simulink model "cubli_XYZ_extensive_simulations"  (R2016a)
settings: Solver=VariableStepAuto  StartTime=0.0  StopTime=10  FixedStep=0.001  RelTol=1e-3
values from neighbouring files (symbols this model uses):
  a = 0.15    [init.m]
  M = 2.5    [init.m]    (also in skew.m = [0 -z y)
  m = 0.204    [init.m]
  s = size(delta_i)    [accessibility_test.m]    (also in observability_test.m = size(delta_i,1))
  state0 = get_equilibrium(0, -pi/4, pi/2, f, state)    [init.m]
undefined symbols (not defined in the file or in its folder): X, Y, Z
libraries: sm_lib x15, nesl_utility x13
(part 2 of 9)

== matlab function cubli_XYZ_extensive_simulations/Cubli/Controller/noninteractive feedback control ==
  data: v input; state input; u output
 function u = nic_fnc(v, state)

th1 = state(1);
th2 = state(2);
th3 = state(3);

th1dot = state(4);
th2dot = state(5);
th3dot = state(6);
qxdot = state(7);
qydot = state(8);
qzdot = state(9);

A = [                                                                                                                  -(11529215046068469760000*(173808361171031714041*cos(th3) - 97421867139278569472*sin(th3)))/(50688073959935957106266099682798465939237*cos(th2)*(cos(th3)^2 + sin(th3)^2)),                                                                                                                  -(11529215046068469760000*(97421867139278569472*cos(th3) - 173808361171031714041*sin(th3)))/(50688073959935957106266099682798465939237*cos(th2)*(cos(th3)^2 + sin(th3)^2)),                                                                                                                                          -(1123197656438253912603716965936891166720000*(cos(th3) - sin(th3)))/(50688073959935957106266099682798465939237*cos(th2)*(cos(th3)^2 + sin(th3)^2))
                                                                                                                           -(11529215046068469760000*(97421867139278569472*cos(th3) + 173808361171031714041*sin(th3)))/(50688073959935957106266099682798465939237*(cos(th3)^2 + sin(th3)^2)),                                                                                                                           -(11529215046068469760000*(173808361171031714041*cos(th3) + 97421867139278569472*sin(th3)))/(50688073959935957106266099682798465939237*(cos(th3)^2 + sin(th3)^2)),                                                                                                                                                   -(1123197656438253912603716965936891166720000*(cos(th3) + sin(th3)))/(50688073959935957106266099682798465939237*(cos(th3)^2 + sin(th3)^2))
 -(11529215046068469760000*(97421867139278569472*sin(th2)*sin(th3) - 173808361171031714041*cos(th3)*sin(th2) + 97421867139278569472*cos(th2)*cos(th3)^2 + 97421867139278569472*cos(th2)*sin(th3)^2))/(50688073959935957106266099682798465939237*(cos(th2)*cos(th3)^2 + cos(th2)*sin(th3)^2)), -(11529215046068469760000*(173808361171031714041*sin(th2)*sin(th3) - 97421867139278569472*cos(th3)*sin(th2) + 97421867139278569472*cos(th2)*cos(th3)^2 + 97421867139278569472*cos(th2)*sin(th3)^2))/(50688073959935957106266099682798465939237*(cos(th2)*cos(th3)^2 + cos(th2)*sin(th3)^2)), -(11529215046068469760000*(97421867139278569472*sin(th2)*sin(th3) - 97421867139278569472*cos(th3)*sin(th2) + 173808361171031714041*cos(th2)*cos(th3)^2 + 173808361171031714041*cos(th2)*sin(th3)^2))/(50688073959935957106266099682798465939237*(cos(th2)*cos(th3)^2 + cos(th2)*sin(th3)^2))];
 
b = [                                                                                                                                                                                                                                                                                                                                                                                                                                                                                                                                                                                                                                                                                                                                                                                                                                                                                                                                                                                                                                                                                                                                                                                                                                                                                                                                                                                                                                                                                                                                                                                                                                                                                                                                                                                                                                                                                                                                                                                                                                                                                                                                                                                                                                                                                                                                                                                                                                                                                                                                                                                                                                                                                                                                                                                                                                                                                                                                                                                                                                                                                                                                                                                                                                                                                                                                                                                                                                                                                                                                                                                                                                                                                                                                                                                                                                                                                                                                                                                                                                                                                                                                                                                                                                                                                                                                                                                                                                                                                                                                                                                                                                                                                                                                                                                                                                                                                                                                                                                                                                                                                                                                                                                                                                                                                                                                                                                                                                                                                                                                                                                                                                                                                                                                                                                                                                                                                                                                                                                                                                                                                                                                                                                                                                                                                                                                                                                                                                                                                                                                                                                                                                                                                                                                                                                                                                                                                                                                                                                                                                                                                                                                                                                                                                                                                                                                                                                                                                                                                                                                                                                                                                                                                                                                                                                                                                                                                                                                                                                                                                                                                                                                                                                                                                                                                                                                                                                                                                                                                                                                                                                                                                                                                                                                                                                           -(11909473891670740540090329827195917399228416*cos(th1)*cos(th3)^3 + 11909473891670740540090329827195917399228416*cos(th1)*sin(th3)^3 - 84663675348499979021291712024873281781760*th2dot^2*cos(th2)*cos(th3)^3 + 37208574363983751213784670214039629987840*th3dot^2*cos(th2)*cos(th3)^3 + 47455100984516227807507041810833651793920*th2dot^2*cos(th2)*cos(th3)^5 - 84663675348499979021291712024873281781760*th2dot^2*cos(th2)*sin(th3)^3 + 37208574363983751213784670214039629987840*th3dot^2*cos(th2)*sin(th3)^3 + 47455100984516227807507041810833651793920*th2dot^2*cos(th2)*sin(th3)^5 - 11909473891670740540090329827195917399228416*cos(th2)*cos(th3)^2*sin(th1) - 1441358891699742679378121702564642609430528*cos(th1)*cos(th3)*sin(th3)^2 - 1441358891699742679378121702564642609430528*cos(th1)*cos(th3)^2*sin(th3) + 6675416391685241609734225764880280004329472*cos(th2)*cos(th3)^4*sin(th1) - 11909473891670740540090329827195917399228416*cos(th2)*sin(th1)*sin(th3)^2 + 6675416391685241609734225764880280004329472*cos(th2)*sin(th1)*sin(th3)^4 + 47455100984516227807507041810833651793920*th1dot^2*cos(th2)^3*cos(th3)^3 - 47455100984516227807507041810833651793920*th1dot^2*cos(th2)^3*cos(th3)^5 - 6675416391685241609734225764880280004329472*cos(th1)*cos(th2)^2*cos(th3)^3 + 47455100984516227807507041810833651793920*th1dot^2*cos(th2)^3*sin(th3)^3 - 47455100984516227807507041810833651793920*th1dot^2*cos(th2)^3*sin(th3)^5 - 6675416391685241609734225764880280004329472*cos(th1)*cos(th2)^2*sin(th3)^3 - 11909473891670740540090329827195917399228416*cos(th1)*cos(th3)^3*sin(th2)^2 - 11909473891670740540090329827195917399228416*cos(th1)*sin(th2)^2*sin(th3)^3 + 10246526620532476593722371596794021806080*th2dot^2*cos(th2)*cos(th3)*sin(th3)^2 + 10246526620532476593722371596794021806080*th2dot^2*cos(th2)*cos(th3)^2*sin(th3) + 37208574363983751213784670214039629987840*th3dot^2*cos(th2)*cos(th3)*sin(th3)^2 + 37208574363983751213784670214039629987840*th3dot^2*cos(th2)*cos(th3)^2*sin(th3) - 47455100984516227807507041810833651793920*th2dot^2*cos(th2)*cos(th3)*sin(th3)^4 - 47455100984516227807507041810833651793920*th2dot^2*cos(th2)*cos(th3)^4*sin(th3) - 6675416391685241609734225764880280004329472*cos(th1)*cos(th2)*cos(th3)^2*sin(th2) + 6675416391685241609734225764880280004329472*cos(th1)*cos(th2)*cos(th3)^4*sin(th2) + 6675416391685241609734225764880280004329472*cos(th1)*cos(th2)*sin(th2)*sin(th3)^2 - 6675416391685241609734225764880280004329472*cos(th1)*cos(th2)*sin(th2)*sin(th3)^4 - 13350832783370483219468451529760560008658944*cos(th2)*cos(th3)*sin(th1)*sin(th3)^3 - 13350832783370483219468451529760560008658944*cos(th2)*cos(th3)^3*sin(th1)*sin(th3) - 795598339977096578581794905915392000000*qxdot*th2dot*cos(th2)*cos(th3)^4 + 795598339977096578581794905915392000000*qxdot*th3dot*cos(th2)*cos(th3)^3 - 1419410730694772925795933922925238500000*qydot*th3dot*cos(th2)*cos(th3)^3 + 1419410730694772925795933922925238500000*qzdot*th2dot*cos(th2)*cos(th3)^2 + 237129818143993776058215849996810503030165*th2dot*th3dot*cos(th2)*cos(th3)^2 - 96329612699727228540810017544592542087840*th2dot*th3dot*cos(th2)*cos(th3)^4 - 1419410730694772925795933922925238500000*qxdot*th3dot*cos(th2)*sin(th3)^3 - 795598339977096578581794905915392000000*qydot*th2dot*cos(th2)*sin(th3)^4 + 795598339977096578581794905915392000000*qydot*th3dot*cos(th2)*sin(th3)^3 + 1419410730694772925795933922925238500000*qzdot*th2dot*cos(th2)*sin(th3)^2 + 237129818143993776058215849996810503030165*th2dot*th3dot*cos(th2)*sin(th3)^2 - 96329612699727228540810017544592542087840*th2dot*th3dot*cos(th2)*sin(th3)^4 - 132914374672993303407380548741622325575680*th1dot^2*cos(th2)^2*cos(th3)^2*sin(th2) + 37208574363983751213784670214039629987840*th1dot^2*cos(th2)*cos(th3)^3*sin(th2)^2 + 170122949036977054621165218955661955563520*th1dot^2*cos(th2)^2*cos(th3)^4*sin(th2) - 47455100984516227807507041810833651793920*th1dot^2*cos(th2)^3*cos(th3)*sin(th3)^2 - 47455100984516227807507041810833651793920*th1dot^2*cos(th2)^3*cos(th3)^2*sin(th3) + 47455100984516227807507041810833651793920*th1dot^2*cos(th2)^3*cos(th3)*sin(th3)^4 + 47455100984516227807507041810833651793920*th1dot^2*cos(th2)^3*cos(th3)^4*sin(th3) + 6675416391685241609734225764880280004329472*cos(th1)*cos(th2)^2*cos(th3)*sin(th3)^2 + 6675416391685241609734225764880280004329472*cos(th1)*cos(th2)^2*cos(th3)^2*sin(th3) + 132914374672993303407380548741622325575680*th1dot^2*cos(th2)^2*sin(th2)*sin(th3)^2 + 37208574363983751213784670214039629987840*th1dot^2*cos(th2)*sin(th2)^2*sin(th3)^3 - 170122949036977054621165218955661955563520*th1dot^2*cos(th2)^2*sin(th2)*sin(th3)^4 + 1441358891699742679378121702564642609430528*cos(th1)*cos(th3)*sin(th2)^2*sin(th3)^2 + 1441358891699742679378121702564642609430528*cos(th1)*cos(th3)^2*sin(th2)^2*sin(th3) + 13350832783370483219468451529760560008658944*cos(th2)*cos(th3)^2*sin(th1)*sin(th3)^2 + 795598339977096578581794905915392000000*qydot*th1dot*cos(th2)^2*cos(th3)^4 - 795598339977096578581794905915392000000*qzdot*th1dot*cos(th2)^2*cos(th3)^2 - 37208574363983751213784670214039629987840*th1dot*th2dot*cos(th2)^2*cos(th3)^3 - 132914374672993303407380548741622325575680*th1dot*th3dot*cos(th2)^2*cos(th3)^2 + 170122949036977054621165218955661955563520*th1dot*th3dot*cos(th2)^2*cos(th3)^4 - 795598339977096578581794905915392000000*qxdot*th1dot*cos(th2)^2*sin(th3)^4 + 795598339977096578581794905915392000000*qzdot*th1dot*cos(th2)^2*sin(th3)^2 + 37208574363983751213784670214039629987840*th1dot*th2dot*cos(th2)^2*sin(th3)^3 + 132914374672993303407380548741622325575680*th1dot*th3dot*cos(th2)^2*sin(th3)^2 - 170122949036977054621165218955661955563520*th1dot*th3dot*cos(th2)^2*sin(th3)^4 + 13350832783370483219468451529760560008658944*cos(th2)*cos(th3)*sin(th1)*sin(th3) + 795598339977096578581794905915392000000*qxdot*th1dot*cos(th2)*cos(th3)^3*sin(th2) + 795598339977096578581794905915392000000*qxdot*th2dot*cos(th2)*cos(th3)*sin(th3)^3 + 795598339977096578581794905915392000000*qxdot*th2dot*cos(th2)*cos(th3)^3*sin(th3) + 795598339977096578581794905915392000000*qxdot*th3dot*cos(th2)*cos(th3)*sin(th3)^2 - 1419410730694772925795933922925238500000*qxdot*th3dot*cos(th2)*cos(th3)^2*sin(th3) - 1419410730694772925795933922925238500000*qydot*th1dot*cos(th2)*cos(th3)^3*sin(th2) + 795598339977096578581794905915392000000*qydot*th2dot*cos(th2)*cos(th3)*sin(th3)^3 + 795598339977096578581794905915392000000*qydot*th2dot*cos(th2)*cos(th3)^3*sin(th3) - 1419410730694772925795933922925238500000*qydot*th3dot*cos(th2)*cos(th3)*sin(th3)^2 + 795598339977096578581794905915392000000*qydot*th3dot*cos(th2)*cos(th3)^2*sin(th3) + 237129818143993776058215849996810503030165*th1dot*th2dot*cos(th2)*cos(th3)^2*sin(th2) - 377930023588260323575621682449028463972490*th1dot*th2dot*cos(th2)*cos(th3)^4*sin(th2) + 74417148727967502427569340428079259975680*th1dot*th3dot*cos(th2)*cos(th3)^3*sin(th2) + 340245898073954109242330437911323911127040*th2dot*th3dot*cos(th2)*cos(th3)*sin(th3)^3 + 340245898073954109242330437911323911127040*th2dot*th3dot*cos(th2)*cos(th3)^3*sin(th3) - 1419410730694772925795933922925238500000*qxdot*th1dot*cos(th2)*sin(th2)*sin(th3)^3 + 795598339977096578581794905915392000000*qydot*th1dot*cos(th2)*sin(th2)*sin(th3)^3 + 237129818143993776058215849996810503030165*th1dot*th2dot*cos(th2)*sin(th2)*sin(th3)^2 - 377930023588260323575621682449028463972490*th1dot*th2dot*cos(th2)*sin(th2)*sin(th3)^4 + 74417148727967502427569340428079259975680*th1dot*th3dot*cos(th2)*sin(th2)*sin(th3)^3 + 37208574363983751213784670214039629987840*th1dot^2*cos(th2)*cos(th3)*sin(th2)^2*sin(th3)^2 + 37208574363983751213784670214039629987840*th1dot^2*cos(th2)*cos(th3)^2*sin(th2)^2*sin(th3) + 795598339977096578581794905915392000000*qxdot*th1dot*cos(th2)^2*cos(th3)*sin(th3)^3 + 795598339977096578581794905915392000000*qxdot*th1dot*cos(th2)^2*cos(th3)^3*sin(th3) - 795598339977096578581794905915392000000*qxdot*th2dot*cos(th2)*cos(th3)^2*sin(th3)^2 - 795598339977096578581794905915392000000*qydot*th1dot*cos(th2)^2*cos(th3)*sin(th3)^3 - 795598339977096578581794905915392000000*qydot*th1dot*cos(th2)^2*cos(th3)^3*sin(th3) - 795598339977096578581794905915392000000*qydot*th2dot*cos(th2)*cos(th3)^2*sin(th3)^2 - 227028978302048662443812837457374237163520*th1dot*th2dot*cos(th2)^2*cos(th3)*sin(th3)^2 + 227028978302048662443812837457374237163520*th1dot*th2dot*cos(th2)^2*cos(th3)^2*sin(th3) + 189820403938064911230028167243334607175680*th1dot*th2dot*cos(th2)^2*cos(th3)*sin(th3)^4 - 189820403938064911230028167243334607175680*th1dot*th2dot*cos(th2)^2*cos(th3)^4*sin(th3) - 192659225399454457081620035089185084175680*th2dot*th3dot*cos(th2)*cos(th3)^2*sin(th3)^2 - 1591196679954193157163589811830784000000*qzdot*th2dot*cos(th2)*cos(th3)*sin(th3) - 265828749345986606814761097483244651151360*th2dot*th3dot*cos(th2)*cos(th3)*sin(th3) - 795598339977096578581794905915392000000*qxdot*th1dot*cos(th2)^2*cos(th3)^2*sin(th3)^2 + 795598339977096578581794905915392000000*qydot*th1dot*cos(th2)^2*cos(th3)^2*sin(th3)^2 - 189820403938064911230028167243334607175680*th1dot*th2dot*cos(th2)^2*cos(th3)^2*sin(th3)^3 + 189820403938064911230028167243334607175680*th1dot*th2dot*cos(th2)^2*cos(th3)^3*sin(th3)^2 + 795598339977096578581794905915392000000*qxdot*th1dot*cos(th2)*cos(th3)*sin(th2)*sin(th3)^2 - 1419410730694772925795933922925238500000*qxdot*th1dot*cos(th2)*cos(th3)^2*sin(th2)*sin(th3) - 1419410730694772925795933922925238500000*qydot*th1dot*cos(th2)*cos(th3)*sin(th2)*sin(th3)^2 + 795598339977096578581794905915392000000*qydot*th1dot*cos(th2)*cos(th3)^2*sin(th2)*sin(th3) + 340245898073954109242330437911323911127040*th1dot*th2dot*cos(th2)*cos(th3)*sin(th2)*sin(th3)^3 + 340245898073954109242330437911323911127040*th1dot*th2dot*cos(th2)*cos(th3)^3*sin(th2)*sin(th3) + 74417148727967502427569340428079259975680*th1dot*th3dot*cos(th2)*cos(th3)*sin(th2)*sin(th3)^2 + 74417148727967502427569340428079259975680*th1dot*th3dot*cos(th2)*cos(th3)^2*sin(th2)*sin(th3) - 755860047176520647151243364898056927944980*th1dot*th2dot*cos(th2)*cos(th3)^2*sin(th2)*sin(th3)^2 - 265828749345986606814761097483244651151360*th1dot*th2dot*cos(th2)*cos(th3)*sin(th2)*sin(th3))/(140800205444266547517405832452217960942325*cos(th2)*(cos(th2)*cos(th3)^2 + cos(th2)*sin(th3)^2)*(cos(th3)^2 + sin(th3)^2))
                                                                                                                                                                                                                                                                                                                                                                                                                                                                                                                                                                                                                                                                                                                                                                                                                                                                                                                                                                                                                                                                                                                                                                                                                                                                                                                                                                                                                                                                                                                                                                                                                                                                                                                                                                                                                                                                                                                                                                                                                                                                                                                                                                                                                                                                                                                                                                                                                                                                                                                                                                                                                                                                                                                                                                                                                                                                                                                                                                                                                                                                                                                                                                                                                                                                                                                                                                                                                                                                                                                                                                                                                                                                                                                                                                                                                                                                                                                                                                                                                                                                                                                                                                                                                                                                                                                                                                                                                                                                                                                                                                                                                                                                                                                                                                                                                                                                                                                                                                                                                                                                                                                                                                                                                                                                                                                                                                                                                                                                                                                                                                                                                                                                                                                                                                                                                                                                                                                                                                                                                                                                                                                                                                                                                                                                                                                                                                                                                                                                                                                                                                                                                                                                                                                                                                                                                                                                                                                                                                                                                                                                                                                                                                                                                                                                                                                                                                                                                                                                                                                                                                                                                                                                                                                                                                                                                                                                                                                                                                                                                                                                                                                                                                                                                                                                                                                                                                                                                                                                                                                                                                                                                                                                                                                                                                    -(6675416391685241609734225764880280004329472*cos(th1)*cos(th3)^3 - 6675416391685241609734225764880280004329472*cos(th1)*sin(th3)^3 - 47455100984516227807507041810833651793920*th2dot^2*cos(th2)*cos(th3)^3 - 37208574363983751213784670214039629987840*th3dot^2*cos(th2)*cos(th3)^3 + 47455100984516227807507041810833651793920*th2dot^2*cos(th2)*cos(th3)^5 + 47455100984516227807507041810833651793920*th2dot^2*cos(th2)*sin(th3)^3 + 37208574363983751213784670214039629987840*th3dot^2*cos(th2)*sin(th3)^3 - 47455100984516227807507041810833651793920*th2dot^2*cos(th2)*sin(th3)^5 - 6675416391685241609734225764880280004329472*cos(th2)*cos(th3)^2*sin(th1) - 6675416391685241609734225764880280004329472*cos(th1)*cos(th3)*sin(th3)^2 + 6675416391685241609734225764880280004329472*cos(th1)*cos(th3)^2*sin(th3) + 6675416391685241609734225764880280004329472*cos(th2)*cos(th3)^4*sin(th1) + 6675416391685241609734225764880280004329472*cos(th2)*sin(th1)*sin(th3)^2 - 6675416391685241609734225764880280004329472*cos(th2)*sin(th1)*sin(th3)^4 + 84663675348499979021291712024873281781760*th1dot^2*cos(th2)^3*cos(th3)^3 - 47455100984516227807507041810833651793920*th1dot^2*cos(th2)^3*cos(th3)^5 - 11909473891670740540090329827195917399228416*cos(th1)*cos(th2)^2*cos(th3)^3 - 84663675348499979021291712024873281781760*th1dot^2*cos(th2)^3*sin(th3)^3 + 47455100984516227807507041810833651793920*th1dot^2*cos(th2)^3*sin(th3)^5 + 11909473891670740540090329827195917399228416*cos(th1)*cos(th2)^2*sin(th3)^3 - 6675416391685241609734225764880280004329472*cos(th1)*cos(th3)^3*sin(th2)^2 + 6675416391685241609734225764880280004329472*cos(th1)*sin(th2)^2*sin(th3)^3 + 47455100984516227807507041810833651793920*th2dot^2*cos(th2)*cos(th3)*sin(th3)^2 - 47455100984516227807507041810833651793920*th2dot^2*cos(th2)*cos(th3)^2*sin(th3) - 37208574363983751213784670214039629987840*th3dot^2*cos(th2)*cos(th3)*sin(th3)^2 + 37208574363983751213784670214039629987840*th3dot^2*cos(th2)*cos(th3)^2*sin(th3) - 47455100984516227807507041810833651793920*th2dot^2*cos(th2)*cos(th3)*sin(th3)^4 + 47455100984516227807507041810833651793920*th2dot^2*cos(th2)*cos(th3)^4*sin(th3) - 11909473891670740540090329827195917399228416*cos(th1)*cos(th2)*cos(th3)^2*sin(th2) + 6675416391685241609734225764880280004329472*cos(th1)*cos(th2)*cos(th3)^4*sin(th2) - 11909473891670740540090329827195917399228416*cos(th1)*cos(th2)*sin(th2)*sin(th3)^2 + 6675416391685241609734225764880280004329472*cos(th1)*cos(th2)*sin(th2)*sin(th3)^4 - 795598339977096578581794905915392000000*qxdot*th2dot*cos(th2)*cos(th3)^4 + 1419410730694772925795933922925238500000*qxdot*th3dot*cos(th2)*cos(th3)^3 - 795598339977096578581794905915392000000*qydot*th3dot*cos(th2)*cos(th3)^3 + 795598339977096578581794905915392000000*qzdot*th2dot*cos(th2)*cos(th3)^2 + 132914374672993303407380548741622325575680*th2dot*th3dot*cos(th2)*cos(th3)^2 - 170122949036977054621165218955661955563520*th2dot*th3dot*cos(th2)*cos(th3)^4 + 795598339977096578581794905915392000000*qxdot*th3dot*cos(th2)*sin(th3)^3 + 795598339977096578581794905915392000000*qydot*th2dot*cos(th2)*sin(th3)^4 - 1419410730694772925795933922925238500000*qydot*th3dot*cos(th2)*sin(th3)^3 - 795598339977096578581794905915392000000*qzdot*th2dot*cos(th2)*sin(th3)^2 - 132914374672993303407380548741622325575680*th2dot*th3dot*cos(th2)*sin(th3)^2 + 170122949036977054621165218955661955563520*th2dot*th3dot*cos(th2)*sin(th3)^4 - 237129818143993776058215849996810503030165*th1dot^2*cos(th2)^2*cos(th3)^2*sin(th2) - 37208574363983751213784670214039629987840*th1dot^2*cos(th2)*cos(th3)^3*sin(th2)^2 + 237129818143993776058215849996810503030165*th1dot^2*cos(th2)^2*cos(th3)^4*sin(th2) - 10246526620532476593722371596794021806080*th1dot^2*cos(th2)^3*cos(th3)*sin(th3)^2 + 10246526620532476593722371596794021806080*th1dot^2*cos(th2)^3*cos(th3)^2*sin(th3) + 47455100984516227807507041810833651793920*th1dot^2*cos(th2)^3*cos(th3)*sin(th3)^4 - 47455100984516227807507041810833651793920*th1dot^2*cos(th2)^3*cos(th3)^4*sin(th3) + 1441358891699742679378121702564642609430528*cos(th1)*cos(th2)^2*cos(th3)*sin(th3)^2 - 1441358891699742679378121702564642609430528*cos(th1)*cos(th2)^2*cos(th3)^2*sin(th3) - 237129818143993776058215849996810503030165*th1dot^2*cos(th2)^2*sin(th2)*sin(th3)^2 + 37208574363983751213784670214039629987840*th1dot^2*cos(th2)*sin(th2)^2*sin(th3)^3 + 237129818143993776058215849996810503030165*th1dot^2*cos(th2)^2*sin(th2)*sin(th3)^4 + 6675416391685241609734225764880280004329472*cos(th1)*cos(th3)*sin(th2)^2*sin(th3)^2 - 6675416391685241609734225764880280004329472*cos(th1)*cos(th3)^2*sin(th2)^2*sin(th3) + 795598339977096578581794905915392000000*qydot*th1dot*cos(th2)^2*cos(th3)^4 - 1419410730694772925795933922925238500000*qzdot*th1dot*cos(th2)^2*cos(th3)^2 + 37208574363983751213784670214039629987840*th1dot*th2dot*cos(th2)^2*cos(th3)^3 - 237129818143993776058215849996810503030165*th1dot*th3dot*cos(th2)^2*cos(th3)^2 + 96329612699727228540810017544592542087840*th1dot*th3dot*cos(th2)^2*cos(th3)^4 + 795598339977096578581794905915392000000*qxdot*th1dot*cos(th2)^2*sin(th3)^4 - 1419410730694772925795933922925238500000*qzdot*th1dot*cos(th2)^2*sin(th3)^2 + 37208574363983751213784670214039629987840*th1dot*th2dot*cos(th2)^2*sin(th3)^3 - 237129818143993776058215849996810503030165*th1dot*th3dot*cos(th2)^2*sin(th3)^2 + 96329612699727228540810017544592542087840*th1dot*th3dot*cos(th2)^2*sin(th3)^4 - 265828749345986606814761097483244651151360*th1dot^2*cos(th2)^2*cos(th3)*sin(th2)*sin(th3) + 13350832783370483219468451529760560008658944*cos(th1)*cos(th2)*cos(th3)*sin(th2)*sin(th3)^3 + 13350832783370483219468451529760560008658944*cos(th1)*cos(th2)*cos(th3)^3*sin(th2)*sin(th3) + 1419410730694772925795933922925238500000*qxdot*th1dot*cos(th2)*cos(th3)^3*sin(th2) - 795598339977096578581794905915392000000*qxdot*th2dot*cos(th2)*cos(th3)*sin(th3)^3 - 795598339977096578581794905915392000000*qxdot*th2dot*cos(th2)*cos(th3)^3*sin(th3) + 1419410730694772925795933922925238500000*qxdot*th3dot*cos(th2)*cos(th3)*sin(th3)^2 + 795598339977096578581794905915392000000*qxdot*th3dot*cos(th2)*cos(th3)^2*sin(th3) - 795598339977096578581794905915392000000*qydot*th1dot*cos(th2)*cos(th3)^3*sin(th2) + 795598339977096578581794905915392000000*qydot*th2dot*cos(th2)*cos(th3)*sin(th3)^3 + 795598339977096578581794905915392000000*qydot*th2dot*cos(th2)*cos(th3)^3*sin(th3) - 795598339977096578581794905915392000000*qydot*th3dot*cos(th2)*cos(th3)*sin(th3)^2 - 1419410730694772925795933922925238500000*qydot*th3dot*cos(th2)*cos(th3)^2*sin(th3) - 1591196679954193157163589811830784000000*qzdot*th1dot*cos(th2)^2*cos(th3)*sin(th3) + 132914374672993303407380548741622325575680*th1dot*th2dot*cos(th2)*cos(th3)^2*sin(th2) - 170122949036977054621165218955661955563520*th1dot*th2dot*cos(th2)*cos(th3)^4*sin(th2) - 74417148727967502427569340428079259975680*th1dot*th3dot*cos(th2)*cos(th3)^3*sin(th2) - 265828749345986606814761097483244651151360*th1dot*th3dot*cos(th2)^2*cos(th3)*sin(th3) + 795598339977096578581794905915392000000*qxdot*th1dot*cos(th2)*sin(th2)*sin(th3)^3 - 1419410730694772925795933922925238500000*qydot*th1dot*cos(th2)*sin(th2)*sin(th3)^3 - 132914374672993303407380548741622325575680*th1dot*th2dot*cos(th2)*sin(th2)*sin(th3)^2 + 170122949036977054621165218955661955563520*th1dot*th2dot*cos(th2)*sin(th2)*sin(th3)^4 + 74417148727967502427569340428079259975680*th1dot*th3dot*cos(th2)*sin(th2)*sin(th3)^3 - 37208574363983751213784670214039629987840*th1dot^2*cos(th2)*cos(th3)*sin(th2)^2*sin(th3)^2 + 37208574363983751213784670214039629987840*th1dot^2*cos(th2)*cos(th3)^2*sin(th2)^2*sin(th3) + 340245898073954109242330437911323911127040*th1dot^2*cos(th2)^2*cos(th3)*sin(th2)*sin(th3)^3 + 340245898073954109242330437911323911127040*th1dot^2*cos(th2)^2*cos(th3)^3*sin(th2)*sin(th3) + 13350832783370483219468451529760560008658944*cos(th1)*cos(th2)*cos(th3)^2*sin(th2)*sin(th3)^2 + 795598339977096578581794905915392000000*qxdot*th1dot*cos(th2)^2*cos(th3)*sin(th3)^3 + 795598339977096578581794905915392000000*qxdot*th1dot*cos(th2)^2*cos(th3)^3*sin(th3) - 795598339977096578581794905915392000000*qxdot*th2dot*cos(th2)*cos(th3)^2*sin(th3)^2 + 795598339977096578581794905915392000000*qydot*th1dot*cos(th2)^2*cos(th3)*sin(th3)^3 + 795598339977096578581794905915392000000*qydot*th1dot*cos(th2)^2*cos(th3)^3*sin(th3) + 795598339977096578581794905915392000000*qydot*th2dot*cos(th2)*cos(th3)^2*sin(th3)^2 + 227028978302048662443812837457374237163520*th1dot*th2dot*cos(th2)^2*cos(th3)*sin(th3)^2 + 227028978302048662443812837457374237163520*th1dot*th2dot*cos(th2)^2*cos(th3)^2*sin(th3) - 189820403938064911230028167243334607175680*th1dot*th2dot*cos(th2)^2*cos(th3)*sin(th3)^4 - 189820403938064911230028167243334607175680*th1dot*th2dot*cos(th2)^2*cos(th3)^4*sin(th3) + 340245898073954109242330437911323911127040*th1dot*th3dot*cos(th2)^2*cos(th3)*sin(th3)^3 + 340245898073954109242330437911323911127040*th1dot*th3dot*cos(th2)^2*cos(th3)^3*sin(th3) - 13350832783370483219468451529760560008658944*cos(th1)*cos(th2)*cos(th3)*sin(th2)*sin(th3) + 474259636287987552116431699993621006060330*th1dot^2*cos(th2)^2*cos(th3)^2*sin(th2)*sin(th3)^2 + 795598339977096578581794905915392000000*qxdot*th1dot*cos(th2)^2*cos(th3)^2*sin(th3)^2 + 795598339977096578581794905915392000000*qydot*th1dot*cos(th2)^2*cos(th3)^2*sin(th3)^2 - 189820403938064911230028167243334607175680*th1dot*th2dot*cos(th2)^2*cos(th3)^2*sin(th3)^3 - 189820403938064911230028167243334607175680*th1dot*th2dot*cos(th2)^2*cos(th3)^3*sin(th3)^2 + 192659225399454457081620035089185084175680*th1dot*th3dot*cos(th2)^2*cos(th3)^2*sin(th3)^2 + 1419410730694772925795933922925238500000*qxdot*th1dot*cos(th2)*cos(th3)*sin(th2)*sin(th3)^2 + 795598339977096578581794905915392000000*qxdot*th1dot*cos(th2)*cos(th3)^2*sin(th2)*sin(th3) - 795598339977096578581794905915392000000*qydot*th1dot*cos(th2)*cos(th3)*sin(th2)*sin(th3)^2 - 1419410730694772925795933922925238500000*qydot*th1dot*cos(th2)*cos(th3)^2*sin(th2)*sin(th3) - 74417148727967502427569340428079259975680*th1dot*th3dot*cos(th2)*cos(th3)*sin(th2)*sin(th3)^2 + 74417148727967502427569340428079259975680*th1dot*th3dot*cos(th2)*cos(th3)^2*sin(th2)*sin(th3))/(140800205444266547517405832452217960942325*(cos(th2)*cos(th3)^2 + cos(th2)*sin(th3)^2)*(cos(th3)^2 + sin(th3)^2))
 (11909473891670740540090329827195917399228416*cos(th1)*cos(th3)^3*sin(th2) - 6675416391685241609734225764880280004329472*cos(th1)*cos(th2)*cos(th3)^4 + 6675416391685241609734225764880280004329472*cos(th1)*cos(th2)*sin(th3)^4 + 11909473891670740540090329827195917399228416*cos(th1)*sin(th2)*sin(th3)^3 + 47455100984516227807507041810833651793920*th2dot^2*cos(th2)^2*cos(th3)^4 - 47455100984516227807507041810833651793920*th1dot^2*cos(th2)^4*cos(th3)^4 - 84663675348499979021291712024873281781760*th2dot^2*cos(th2)^2*cos(th3)^6 + 84663675348499979021291712024873281781760*th1dot^2*cos(th2)^4*cos(th3)^6 + 6675416391685241609734225764880280004329472*cos(th1)*cos(th2)^3*cos(th3)^4 - 47455100984516227807507041810833651793920*th2dot^2*cos(th2)^2*sin(th3)^4 + 47455100984516227807507041810833651793920*th1dot^2*cos(th2)^4*sin(th3)^4 + 84663675348499979021291712024873281781760*th2dot^2*cos(th2)^2*sin(th3)^6 - 84663675348499979021291712024873281781760*th1dot^2*cos(th2)^4*sin(th3)^6 + 6675416391685241609734225764880280004329472*cos(th2)^2*cos(th3)^3*sin(th1) - 11909473891670740540090329827195917399228416*cos(th1)*cos(th3)^3*sin(th2)^3 - 6675416391685241609734225764880280004329472*cos(th1)*cos(th2)^3*sin(th3)^4 - 11909473891670740540090329827195917399228416*cos(th2)^2*cos(th3)^5*sin(th1) - 6675416391685241609734225764880280004329472*cos(th2)^2*sin(th1)*sin(th3)^3 - 11909473891670740540090329827195917399228416*cos(th1)*sin(th2)^3*sin(th3)^3 + 11909473891670740540090329827195917399228416*cos(th2)^2*sin(th1)*sin(th3)^5 - 84663675348499979021291712024873281781760*th2dot^2*cos(th2)*cos(th3)^3*sin(th2) + 37208574363983751213784670214039629987840*th3dot^2*cos(th2)*cos(th3)^3*sin(th2) + 47455100984516227807507041810833651793920*th2dot^2*cos(th2)*cos(th3)^5*sin(th2) - 84663675348499979021291712024873281781760*th2dot^2*cos(th2)*sin(th2)*sin(th3)^3 + 37208574363983751213784670214039629987840*th3dot^2*cos(th2)*sin(th2)*sin(th3)^3 + 47455100984516227807507041810833651793920*th2dot^2*cos(th2)*sin(th2)*sin(th3)^5 - 11909473891670740540090329827195917399228416*cos(th2)*cos(th3)^2*sin(th1)*sin(th2) - 1441358891699742679378121702564642609430528*cos(th1)*cos(th3)*sin(th2)*sin(th3)^2 - 1441358891699742679378121702564642609430528*cos(th1)*cos(th3)^2*sin(th2)*sin(th3) + 6675416391685241609734225764880280004329472*cos(th2)*cos(th3)^4*sin(th1)*sin(th2) - 11909473891670740540090329827195917399228416*cos(th2)*sin(th1)*sin(th2)*sin(th3)^2 + 6675416391685241609734225764880280004329472*cos(th2)*sin(th1)*sin(th2)*sin(th3)^4 + 37208574363983751213784670214039629987840*th1dot^2*cos(th2)*cos(th3)^3*sin(th2)^3 + 180369475657509531214887590552455977369600*th1dot^2*cos(th2)^3*cos(th3)^3*sin(th2) - 143160901293525780001102920338416347381760*th1dot^2*cos(th2)^3*cos(th3)^5*sin(th2) - 6675416391685241609734225764880280004329472*cos(th1)*cos(th2)*cos(th3)^2*sin(th2)^2 + 13350832783370483219468451529760560008658944*cos(th1)*cos(th2)*cos(th3)^4*sin(th2)^2 - 11909473891670740540090329827195917399228416*cos(th1)*cos(th2)^2*cos(th3)^5*sin(th2) + 37208574363983751213784670214039629987840*th1dot^2*cos(th2)*sin(th2)^3*sin(th3)^3 + 180369475657509531214887590552455977369600*th1dot^2*cos(th2)^3*sin(th2)*sin(th3)^3 - 143160901293525780001102920338416347381760*th1dot^2*cos(th2)^3*sin(th2)*sin(th3)^5 + 6675416391685241609734225764880280004329472*cos(th1)*cos(th2)*sin(th2)^2*sin(th3)^2 + 6675416391685241609734225764880280004329472*cos(th2)^2*cos(th3)*sin(th1)*sin(th3)^2 - 6675416391685241609734225764880280004329472*cos(th2)^2*cos(th3)^2*sin(th1)*sin(th3) - 13350832783370483219468451529760560008658944*cos(th1)*cos(th2)*sin(th2)^2*sin(th3)^4 + 1441358891699742679378121702564642609430528*cos(th1)*cos(th3)*sin(th2)^3*sin(th3)^2 + 1441358891699742679378121702564642609430528*cos(th1)*cos(th3)^2*sin(th2)^3*sin(th3) - 11909473891670740540090329827195917399228416*cos(th1)*cos(th2)^2*sin(th2)*sin(th3)^5 - 11909473891670740540090329827195917399228416*cos(th2)^2*cos(th3)*sin(th1)*sin(th3)^4 + 11909473891670740540090329827195917399228416*cos(th2)^2*cos(th3)^4*sin(th1)*sin(th3) + 1419410730694772925795933922925238500000*qxdot*th2dot*cos(th2)^2*cos(th3)^5 - 795598339977096578581794905915392000000*qxdot*th3dot*cos(th2)^2*cos(th3)^4 - 1419410730694772925795933922925238500000*qydot*th1dot*cos(th2)^3*cos(th3)^5 + 795598339977096578581794905915392000000*qydot*th3dot*cos(th2)^2*cos(th3)^4 + 795598339977096578581794905915392000000*qzdot*th1dot*cos(th2)^3*cos(th3)^3 - 795598339977096578581794905915392000000*qzdot*th2dot*cos(th2)^2*cos(th3)^3 - 140800205444266547517405832452217960942325*th1dot*th2dot*cos(th2)^3*cos(th3)^4 + 132914374672993303407380548741622325575680*th1dot*th3dot*cos(th2)^3*cos(th3)^3 - 132914374672993303407380548741622325575680*th2dot*th3dot*cos(th2)^2*cos(th3)^3 - 95705800309009552193595878527582695587840*th1dot*th3dot*cos(th2)^3*cos(th3)^5 + 95705800309009552193595878527582695587840*th2dot*th3dot*cos(th2)^2*cos(th3)^5 - 1419410730694772925795933922925238500000*qxdot*th1dot*cos(th2)^3*sin(th3)^5 - 795598339977096578581794905915392000000*qxdot*th3dot*cos(th2)^2*sin(th3)^4 - 1419410730694772925795933922925238500000*qydot*th2dot*cos(th2)^2*sin(th3)^5 + 795598339977096578581794905915392000000*qydot*th3dot*cos(th2)^2*sin(th3)^4 + 795598339977096578581794905915392000000*qzdot*th1dot*cos(th2)^3*sin(th3)^3 + 795598339977096578581794905915392000000*qzdot*th2dot*cos(th2)^2*sin(th3)^3 - 140800205444266547517405832452217960942325*th1dot*th2dot*cos(th2)^3*sin(th3)^4 + 132914374672993303407380548741622325575680*th1dot*th3dot*cos(th2)^3*sin(th3)^3 + 132914374672993303407380548741622325575680*th2dot*th3dot*cos(th2)^2*sin(th3)^3 - 95705800309009552193595878527582695587840*th1dot*th3dot*cos(th2)^3*sin(th3)^5 - 95705800309009552193595878527582695587840*th2dot*th3dot*cos(th2)^2*sin(th3)^5 - 132914374672993303407380548741622325575680*th1dot^2*cos(th2)^2*cos(th3)^2*sin(th2)^2 + 170122949036977054621165218955661955563520*th1dot^2*cos(th2)^2*cos(th3)^4*sin(th2)^2 + 84663675348499979021291712024873281781760*th2dot^2*cos(th2)^2*cos(th3)^2*sin(th3)^4 - 84663675348499979021291712024873281781760*th2dot^2*cos(th2)^2*cos(th3)^4*sin(th3)^2 - 84663675348499979021291712024873281781760*th1dot^2*cos(th2)^4*cos(th3)^2*sin(th3)^4 + 84663675348499979021291712024873281781760*th1dot^2*cos(th2)^4*cos(th3)^4*sin(th3)^2 + 132914374672993303407380548741622325575680*th1dot^2*cos(th2)^2*sin(th2)^2*sin(th3)^2 - 170122949036977054621165218955661955563520*th1dot^2*cos(th2)^2*sin(th2)^2*sin(th3)^4 + 23818947783341481080180659654391834798456832*cos(th2)^2*cos(th3)^2*sin(th1)*sin(th3)^3 - 23818947783341481080180659654391834798456832*cos(th2)^2*cos(th3)^3*sin(th1)*sin(th3)^2 + 10246526620532476593722371596794021806080*th2dot^2*cos(th2)*cos(th3)*sin(th2)*sin(th3)^2 + 10246526620532476593722371596794021806080*th2dot^2*cos(th2)*cos(th3)^2*sin(th2)*sin(th3) + 37208574363983751213784670214039629987840*th3dot^2*cos(th2)*cos(th3)*sin(th2)*sin(th3)^2 + 37208574363983751213784670214039629987840*th3dot^2*cos(th2)*cos(th3)^2*sin(th2)*sin(th3) - 47455100984516227807507041810833651793920*th2dot^2*cos(th2)*cos(th3)*sin(th2)*sin(th3)^4 - 47455100984516227807507041810833651793920*th2dot^2*cos(th2)*cos(th3)^4*sin(th2)*sin(th3) - 13350832783370483219468451529760560008658944*cos(th2)*cos(th3)*sin(th1)*sin(th2)*sin(th3)^3 - 13350832783370483219468451529760560008658944*cos(th2)*cos(th3)^3*sin(th1)*sin(th2)*sin(th3) - 795598339977096578581794905915392000000*qxdot*th2dot*cos(th2)*cos(th3)^4*sin(th2) + 795598339977096578581794905915392000000*qxdot*th3dot*cos(th2)*cos(th3)^3*sin(th2) - 1419410730694772925795933922925238500000*qydot*th3dot*cos(th2)*cos(th3)^3*sin(th2) + 1419410730694772925795933922925238500000*qzdot*th2dot*cos(th2)*cos(th3)^2*sin(th2) + 237129818143993776058215849996810503030165*th2dot*th3dot*cos(th2)*cos(th3)^2*sin(th2) - 96329612699727228540810017544592542087840*th2dot*th3dot*cos(th2)*cos(th3)^4*sin(th2) - 1419410730694772925795933922925238500000*qxdot*th3dot*cos(th2)*sin(th2)*sin(th3)^3 - 795598339977096578581794905915392000000*qydot*th2dot*cos(th2)*sin(th2)*sin(th3)^4 + 795598339977096578581794905915392000000*qydot*th3dot*cos(th2)*sin(th2)*sin(th3)^3 + 1419410730694772925795933922925238500000*qzdot*th2dot*cos(th2)*sin(th2)*sin(th3)^2 + 237129818143993776058215849996810503030165*th2dot*th3dot*cos(th2)*sin(th2)*sin(th3)^2 - 96329612699727228540810017544592542087840*th2dot*th3dot*cos(th2)*sin(th2)*sin(th3)^4 + 37208574363983751213784670214039629987840*th1dot^2*cos(th2)*cos(th3)*sin(th2)^3*sin(th3)^2 + 37208574363983751213784670214039629987840*th1dot^2*cos(th2)*cos(th3)^2*sin(th2)^3*sin(th3) + 85459273688477075599873506930788673781760*th1dot^2*cos(th2)^3*cos(th3)*sin(th2)*sin(th3)^2 + 85459273688477075599873506930788673781760*th1dot^2*cos(th2)^3*cos(th3)^2*sin(th2)*sin(th3) - 48250699324493324386088836716749043793920*th1dot^2*cos(th2)^3*cos(th3)*sin(th2)*sin(th3)^4 - 48250699324493324386088836716749043793920*th1dot^2*cos(th2)^3*cos(th3)^4*sin(th2)*sin(th3) + 13350832783370483219468451529760560008658944*cos(th1)*cos(th2)^2*cos(th3)*sin(th2)*sin(th3)^2 + 13350832783370483219468451529760560008658944*cos(th1)*cos(th2)^2*cos(th3)^2*sin(th2)*sin(th3) - 11909473891670740540090329827195917399228416*cos(th1)*cos(th2)^2*cos(th3)*sin(th2)*sin(th3)^4 - 11909473891670740540090329827195917399228416*cos(th1)*cos(th2)^2*cos(th3)^4*sin(th2)*sin(th3) + 13350832783370483219468451529760560008658944*cos(th2)*cos(th3)^2*sin(th1)*sin(th2)*sin(th3)^2 + 795598339977096578581794905915392000000*qxdot*th1dot*cos(th2)*cos(th3)^3*sin(th2)^2 - 795598339977096578581794905915392000000*qxdot*th1dot*cos(th2)^2*cos(th3)^4*sin(th2) - 1419410730694772925795933922925238500000*qxdot*th1dot*cos(th2)^3*cos(th3)^4*sin(th3) + 1419410730694772925795933922925238500000*qxdot*th2dot*cos(th2)^2*cos(th3)*sin(th3)^4 - 1419410730694772925795933922925238500000*qydot*th1dot*cos(th2)*cos(th3)^3*sin(th2)^2 + 1591196679954193157163589811830784000000*qydot*th1dot*cos(th2)^2*cos(th3)^4*sin(th2) - 1419410730694772925795933922925238500000*qydot*th1dot*cos(th2)^3*cos(th3)*sin(th3)^4 - 1419410730694772925795933922925238500000*qydot*th2dot*cos(th2)^2*cos(th3)^4*sin(th3) - 795598339977096578581794905915392000000*qzdot*th1dot*cos(th2)^2*cos(th3)^2*sin(th2) + 795598339977096578581794905915392000000*qzdot*th1dot*cos(th2)^3*cos(th3)*sin(th3)^2 + 795598339977096578581794905915392000000*qzdot*th1dot*cos(th2)^3*cos(th3)^2*sin(th3) - 795598339977096578581794905915392000000*qzdot*th2dot*cos(th2)^2*cos(th3)*sin(th3)^2 + 795598339977096578581794905915392000000*qzdot*th2dot*cos(th2)^2*cos(th3)^2*sin(th3) + 237129818143993776058215849996810503030165*th1dot*th2dot*cos(th2)*cos(th3)^2*sin(th2)^2 - 170122949036977054621165218955661955563520*th1dot*th2dot*cos(th2)^2*cos(th3)^3*sin(th2) - 132914374672993303407380548741622325575680*th1dot*th3dot*cos(th2)^2*cos(th3)^2*sin(th2) - 377930023588260323575621682449028463972490*th1dot*th2dot*cos(th2)*cos(th3)^4*sin(th2)^2 + 74417148727967502427569340428079259975680*th1dot*th3dot*cos(th2)*cos(th3)^3*sin(th2)^2 + 95705800309009552193595878527582695587840*th1dot*th2dot*cos(th2)^2*cos(th3)^5*sin(th2) - 189820403938064911230028167243334607175680*th1dot*th2dot*cos(th2)^3*cos(th3)*sin(th3)^3 - 189820403938064911230028167243334607175680*th1dot*th2dot*cos(th2)^3*cos(th3)^3*sin(th3) + 170122949036977054621165218955661955563520*th1dot*th3dot*cos(th2)^2*cos(th3)^4*sin(th2) + 132914374672993303407380548741622325575680*th1dot*th3dot*cos(th2)^3*cos(th3)*sin(th3)^2 + 132914374672993303407380548741622325575680*th1dot*th3dot*cos(th2)^3*cos(th3)^2*sin(th3) - 132914374672993303407380548741622325575680*th2dot*th3dot*cos(th2)^2*cos(th3)*sin(th3)^2 + 132914374672993303407380548741622325575680*th2dot*th3dot*cos(th2)^2*cos(th3)^2*sin(th3) + 338654701393999916085166848099493127127040*th1dot*th2dot*cos(th2)^3*cos(th3)*sin(th3)^5 + 338654701393999916085166848099493127127040*th1dot*th2dot*cos(th2)^3*cos(th3)^5*sin(th3) - 95705800309009552193595878527582695587840*th1dot*th3dot*cos(th2)^3*cos(th3)*sin(th3)^4 - 95705800309009552193595878527582695587840*th1dot*th3dot*cos(th2)^3*cos(th3)^4*sin(th3) + 95705800309009552193595878527582695587840*th2dot*th3dot*cos(th2)^2*cos(th3)*sin(th3)^4 - 95705800309009552193595878527582695587840*th2dot*th3dot*cos(th2)^2*cos(th3)^4*sin(th3) - 1419410730694772925795933922925238500000*qxdot*th1dot*cos(th2)*sin(th2)^2*sin(th3)^3 - 1591196679954193157163589811830784000000*qxdot*th1dot*cos(th2)^2*sin(th2)*sin(th3)^4 + 795598339977096578581794905915392000000*qydot*th1dot*cos(th2)*sin(th2)^2*sin(th3)^3 + 795598339977096578581794905915392000000*qydot*th1dot*cos(th2)^2*sin(th2)*sin(th3)^4 + 795598339977096578581794905915392000000*qzdot*th1dot*cos(th2)^2*sin(th2)*sin(th3)^2 + 237129818143993776058215849996810503030165*th1dot*th2dot*cos(th2)*sin(th2)^2*sin(th3)^2 + 170122949036977054621165218955661955563520*th1dot*th2dot*cos(th2)^2*sin(th2)*sin(th3)^3 + 132914374672993303407380548741622325575680*th1dot*th3dot*cos(th2)^2*sin(th2)*sin(th3)^2 - 377930023588260323575621682449028463972490*th1dot*th2dot*cos(th2)*sin(th2)^2*sin(th3)^4 + 74417148727967502427569340428079259975680*th1dot*th3dot*cos(th2)*sin(th2)^2*sin(th3)^3 - 95705800309009552193595878527582695587840*th1dot*th2dot*cos(th2)^2*sin(th2)*sin(th3)^5 - 170122949036977054621165218955661955563520*th1dot*th3dot*cos(th2)^2*sin(th2)*sin(th3)^4 + 13350832783370483219468451529760560008658944*cos(th2)*cos(th3)*sin(th1)*sin(th2)*sin(th3) - 191411600618019104387191757055165391175680*th1dot^2*cos(th2)^3*cos(th3)^2*sin(th2)*sin(th3)^3 - 191411600618019104387191757055165391175680*th1dot^2*cos(th2)^3*cos(th3)^3*sin(th2)*sin(th3)^2 - 23818947783341481080180659654391834798456832*cos(th1)*cos(th2)^2*cos(th3)^2*sin(th2)*sin(th3)^3 - 23818947783341481080180659654391834798456832*cos(th1)*cos(th2)^2*cos(th3)^3*sin(th2)*sin(th3)^2 - 2838821461389545851591867845850477000000*qxdot*th1dot*cos(th2)^3*cos(th3)^2*sin(th3)^3 + 2838821461389545851591867845850477000000*qxdot*th2dot*cos(th2)^2*cos(th3)^3*sin(th3)^2 - 1591196679954193157163589811830784000000*qxdot*th3dot*cos(th2)^2*cos(th3)^2*sin(th3)^2 - 2838821461389545851591867845850477000000*qydot*th1dot*cos(th2)^3*cos(th3)^3*sin(th3)^2 - 2838821461389545851591867845850477000000*qydot*th2dot*cos(th2)^2*cos(th3)^2*sin(th3)^3 + 1591196679954193157163589811830784000000*qydot*th3dot*cos(th2)^2*cos(th3)^2*sin(th3)^2 - 281600410888533095034811664904435921884650*th1dot*th2dot*cos(th2)^3*cos(th3)^2*sin(th3)^2 + 677309402787999832170333696198986254254080*th1dot*th2dot*cos(th2)^3*cos(th3)^3*sin(th3)^3 - 191411600618019104387191757055165391175680*th1dot*th3dot*cos(th2)^3*cos(th3)^2*sin(th3)^3 - 191411600618019104387191757055165391175680*th1dot*th3dot*cos(th2)^3*cos(th3)^3*sin(th3)^2 - 191411600618019104387191757055165391175680*th2dot*th3dot*cos(th2)^2*cos(th3)^2*sin(th3)^3 + 191411600618019104387191757055165391175680*th2dot*th3dot*cos(th2)^2*cos(th3)^3*sin(th3)^2 + 795598339977096578581794905915392000000*qxdot*th2dot*cos(th2)*cos(th3)*sin(th2)*sin(th3)^3 + 795598339977096578581794905915392000000*qxdot*th2dot*cos(th2)*cos(th3)^3*sin(th2)*sin(th3) + 795598339977096578581794905915392000000*qxdot*th3dot*cos(th2)*cos(th3)*sin(th2)*sin(th3)^2 - 1419410730694772925795933922925238500000*qxdot*th3dot*cos(th2)*cos(th3)^2*sin(th2)*sin(th3) + 795598339977096578581794905915392000000*qydot*th2dot*cos(th2)*cos(th3)*sin(th2)*sin(th3)^3 + 795598339977096578581794905915392000000*qydot*th2dot*cos(th2)*cos(th3)^3*sin(th2)*sin(th3) - 1419410730694772925795933922925238500000*qydot*th3dot*cos(th2)*cos(th3)*sin(th2)*sin(th3)^2 + 795598339977096578581794905915392000000*qydot*th3dot*cos(th2)*cos(th3)^2*sin(th2)*sin(th3) - 265828749345986606814761097483244651151360*th1dot*th2dot*cos(th2)*cos(th3)*sin(th2)^2*sin(th3) + 340245898073954109242330437911323911127040*th2dot*th3dot*cos(th2)*cos(th3)*sin(th2)*sin(th3)^3 + 340245898073954109242330437911323911127040*th2dot*th3dot*cos(th2)*cos(th3)^3*sin(th2)*sin(th3) + 795598339977096578581794905915392000000*qxdot*th1dot*cos(th2)*cos(th3)*sin(th2)^2*sin(th3)^2 - 1419410730694772925795933922925238500000*qxdot*th1dot*cos(th2)*cos(th3)^2*sin(th2)^2*sin(th3) + 795598339977096578581794905915392000000*qxdot*th1dot*cos(th2)^2*cos(th3)*sin(th2)*sin(th3)^3 + 795598339977096578581794905915392000000*qxdot*th1dot*cos(th2)^2*cos(th3)^3*sin(th2)*sin(th3) - 795598339977096578581794905915392000000*qxdot*th2dot*cos(th2)*cos(th3)^2*sin(th2)*sin(th3)^2 - 1419410730694772925795933922925238500000*qydot*th1dot*cos(th2)*cos(th3)*sin(th2)^2*sin(th3)^2 + 795598339977096578581794905915392000000*qydot*th1dot*cos(th2)*cos(th3)^2*sin(th2)^2*sin(th3) - 795598339977096578581794905915392000000*qydot*th1dot*cos(th2)^2*cos(th3)*sin(th2)*sin(th3)^3 - 795598339977096578581794905915392000000*qydot*th1dot*cos(th2)^2*cos(th3)^3*sin(th2)*sin(th3) - 795598339977096578581794905915392000000*qydot*th2dot*cos(th2)*cos(th3)^2*sin(th2)*sin(th3)^2 - 359943352975041965851193386198996562739200*th1dot*th2dot*cos(th2)^2*cos(th3)*sin(th2)*sin(th3)^2 + 359943352975041965851193386198996562739200*th1dot*th2dot*cos(th2)^2*cos(th3)^2*sin(th2)*sin(th3) + 340245898073954109242330437911323911127040*th1dot*th2dot*cos(th2)*cos(th3)*sin(th2)^2*sin(th3)^3 + 340245898073954109242330437911323911127040*th1dot*th2dot*cos(th2)*cos(th3)^3*sin(th2)^2*sin(th3) + 74417148727967502427569340428079259975680*th1dot*th3dot*cos(th2)*cos(th3)*sin(th2)^2*sin(th3)^2 + 74417148727967502427569340428079259975680*th1dot*th3dot*cos(th2)*cos(th3)^2*sin(th2)^2*sin(th3) + 285526204247074463423624045770917302763520*th1dot*th2dot*cos(th2)^2*cos(th3)*sin(th2)*sin(th3)^4 - 285526204247074463423624045770917302763520*th1dot*th2dot*cos(th2)^2*cos(th3)^4*sin(th2)*sin(th3) - 192659225399454457081620035089185084175680*th2dot*th3dot*cos(th2)*cos(th3)^2*sin(th2)*sin(th3)^2 - 1591196679954193157163589811830784000000*qzdot*th2dot*cos(th2)*cos(th3)*sin(th2)*sin(th3) - 265828749345986606814761097483244651151360*th2dot*th3dot*cos(th2)*cos(th3)*sin(th2)*sin(th3) - 2386795019931289735745384717746176000000*qxdot*th1dot*cos(th2)^2*cos(th3)^2*sin(th2)*sin(th3)^2 + 2386795019931289735745384717746176000000*qydot*th1dot*cos(th2)^2*cos(th3)^2*sin(th2)*sin(th3)^2 - 755860047176520647151243364898056927944980*th1dot*th2dot*cos(th2)*cos(th3)^2*sin(th2)^2*sin(th3)^2 - 381232004556084015617219924298499998351360*th1dot*th2dot*cos(th2)^2*cos(th3)^2*sin(th2)*sin(th3)^3 + 381232004556084015617219924298499998351360*th1dot*th2dot*cos(th2)^2*cos(th3)^3*sin(th2)*sin(th3)^2)/(140800205444266547517405832452217960942325*(cos(th2)^2*cos(th3)^4 + cos(th2)^2*sin(th3)^4 + 2*cos(th2)^2*cos(th3)^2*sin(th3)^2))];

u = -A \ b + A \ v;
end
